simulink model "FM"  (R2020b)
settings: Solver=VariableStepAuto  StartTime=0.0  StopTime=0.005  RelTol=1e-3
libraries: dsparch4 x1, commsynccomp2 x1
settings Model: Creator=LENOVO  LastModifiedBy=LENOVO

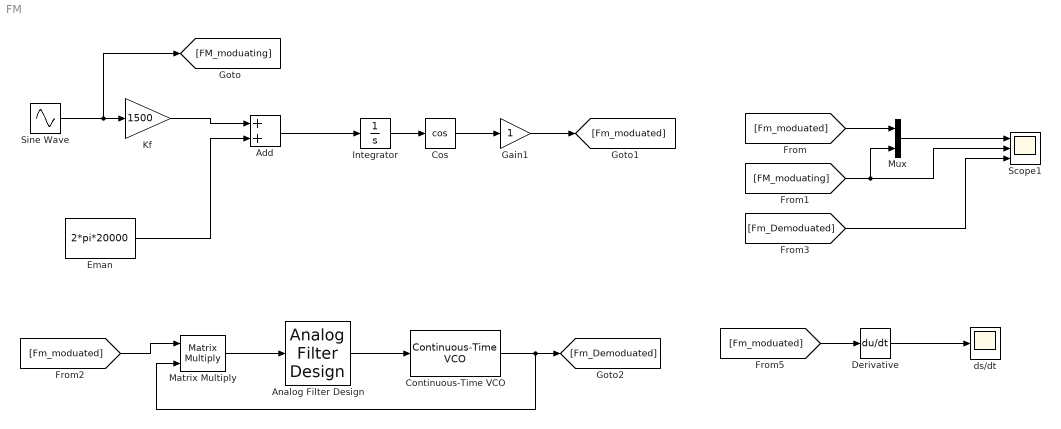
== system FM ==
  Add : Sum
  Analog Filter Design : dsparch4/Analog Filter Design  method=Butterworth  filttype=Lowpass  N=8  Wlo=30  Whi=80  Rp=2  Rs=40
  Continuous-Time VCO : commsynccomp2/Continuous-Time VCO  Ac=1  Fc=10  Kc=1  Ph=0
      settings: SourceProductBaseCode=CM
  Cos : Trigonometry  Operator=cos
  Derivative : Derivative
  Eman : Constant  Value=2*pi*20000
  Gain1 : Gain
  Integrator : Integrator
  Kf : Gain  Gain=1500
  Matrix Multiply : Product  Multiplication=Matrix(*)
  Mux : Mux  Inputs=2
  Scope1 : Scope  NumInputPorts=3
  Sine Wave : Sin  Amplitude=2  Frequency=1000*pi  SampleTime=0
  ds/dt : Scope
  wires:
  Sine Wave/1 -> Kf/1, [FM_moduating]
  Kf/1 -> Add/1
  Eman/1 -> Add/2
  Add/1 -> Integrator/1
  Integrator/1 -> Cos/1
  Cos/1 -> Gain1/1
  Gain1/1 -> [Fm_moduated]
  [Fm_moduated] -> Matrix Multiply/1
  Matrix Multiply/1 -> Analog Filter Design/1
  Analog Filter Design/1 -> Continuous-Time VCO/1
  Continuous-Time VCO/1 -> Matrix Multiply/2, [Fm_Demoduated]
  [Fm_moduated] -> Derivative/1
  Derivative/1 -> ds/dt/1
  [Fm_Demoduated] -> Scope1/3
  [Fm_moduated] -> Mux/1
  [FM_moduating] -> Mux/2, Scope1/2
  Mux/1 -> Scope1/1
